simulink model "mass_spring_3031"  (R2018b)
settings: Solver=FixedStepAuto  StartTime=0.0  StopTime=10.0  RelTol=1e-3
values from neighbouring files (symbols this model uses):
  b = 12    [mass_spring.m]
  f = 8    [mass_spring.m]
  k = 16    [mass_spring.m]
  m = 2    [mass_spring.m]
  x0 = 4    [mass_spring.m]
settings Model: Creator=student  LastModifiedBy=student
settings OptimizationCC: DefaultParameterBehavior=Inlined  UseDivisionForNetSlopeComputation=on  UseFloatMulNetSlope=on  InlineInvariantSignals=on  PassReuseOutputArgsAs=Individual arguments  ZeroExternalMemoryAtStartup=off  ZeroInternalMemoryAtStartup=off  NoFixptDivByZeroProtection=on  EfficientFloat2IntCast=on  LifeSpan=1  OptimizeBlockOrder=speed  DifferentSizesBufferReuse=on
settings DebuggingCC: ParameterTunabilityLossMsg=error
settings HardwareCC: ProdBitPerPointer=32  ProdBitPerSizeT=32  ProdBitPerPtrDiffT=32  ProdWordSize=32  ProdLongLongMode=on  ProdHWDeviceType=Intel->x86-32 (Windows32)
settings SFSimCC: MATLABDynamicMemAlloc=off
settings RTWCC: SystemTargetFile=ert.tlc  TemplateMakefile=ert_default_tmf  GenerateReport=on  IncludeHyperlinkInReport=on  LaunchReport=on  GenerateTraceInfo=on  GenerateTraceReport=on  GenerateTraceReportSl=on  GenerateTraceReportSf=on  GenerateTraceReportEml=on  GenerateCodeMetricsReport=on
settings CodeAppCC: ForceParamTrailComments=on  IgnoreCustomStorageClasses=off  OperatorAnnotations=on  SimulinkDataObjDesc=on  SFDataObjDesc=on  CustomSymbolStrGlobalVar=rt$N$M  CustomSymbolStrType=$N$M  CustomSymbolStrFcn=$N$M$F  CustomSymbolStrMacro=$N$M  InsertBlockDesc=on
settings ERTTargetCC: TargetLangStandard=C99 (ISO)  GenerateSampleERTMain=on  IncludeMdlTerminateFcn=off  CombineSignalStateStructs=on  SupportComplex=off  SupportContinuousTime=on  InlinedParameterPlacement=NonHierarchical  ERTCustomFileTemplate=example_file_process.tlc  ERTFilePackagingFormat=CompactWithDataFile

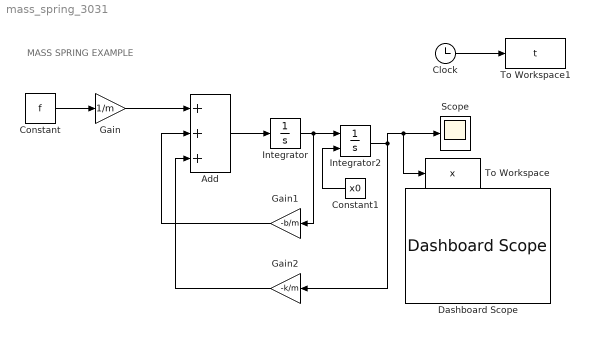
== system mass_spring_3031 ==
  note: MASS SPRING EXAMPLE
  Add : Sum  Inputs=+++
  Clock : Clock
  Constant : Constant  Value=f
  Constant1 : Constant  Value=x0
  Dashboard Scope : DashboardScope  WebBlockId=14
  Gain : Gain  Gain=1/m
  Gain1 : Gain  Gain=-b/m
  Gain2 : Gain  Gain=-k/m
  Integrator : Integrator
  Integrator2 : Integrator  InitialConditionSource=external  AbsoluteTolerance=array
  Scope : Scope
  To Workspace : ToWorkspace  VariableName=x  SaveFormat=Timeseries  SampleTime=-1
  To Workspace1 : ToWorkspace  VariableName=t  SaveFormat=Timeseries  SampleTime=-1
  wires:
  Constant/1 -> Gain/1
  Gain/1 -> Add/1
  Add/1 -> Integrator/1
  Integrator/1 -> Gain1/1, Integrator2/1
  Integrator2/1 -> To Workspace/1, Scope/1, Gain2/1
  Gain2/1 -> Add/3
  Gain1/1 -> Add/2
  Constant1/1 -> Integrator2/2
  Clock/1 -> To Workspace1/1
